simulink model "pll_type2_noise"  (Simulink 6.6)
settings: Solver=VariableStepDiscrete  StartTime=0.0  StopTime=150  RelTol=1e-3
PreLoadFcn:
  | Fs = 1000;
StopFcn:
  | figure(17)
  | hold off
  | plot(Vss_nom,'b');
  | hold on
  | plot(Vss,'r');
  | legend('Centre SS', 'Adj. SS',0);
  | 
  | doFFTplot(Fs, [Vref(round(length(Vref)*0.9):end), Vsyn(round(length(Vsyn)*0.9):end)], ['Input'; 'Synth'], 1, 18, 'hann');
  | 
  | 
  | figure(19)
  | hold off
  | plot(Vref,'b-o');
  | hold on
  | plot(Vsyn,'r-o');
  | plot(zeros(1,length(Vref)),'k--');
  | axis([0 length(Vref) -(max(abs(Vref))*1.2) (max(abs(Vref))*1.2)]);
  | legend('Input','Output',1)
libraries: xbsIndex_r4 x19, dspsrcs4 x1, simulink x1
settings Model: Creator=lcrockett  LastModifiedBy=lcrockett

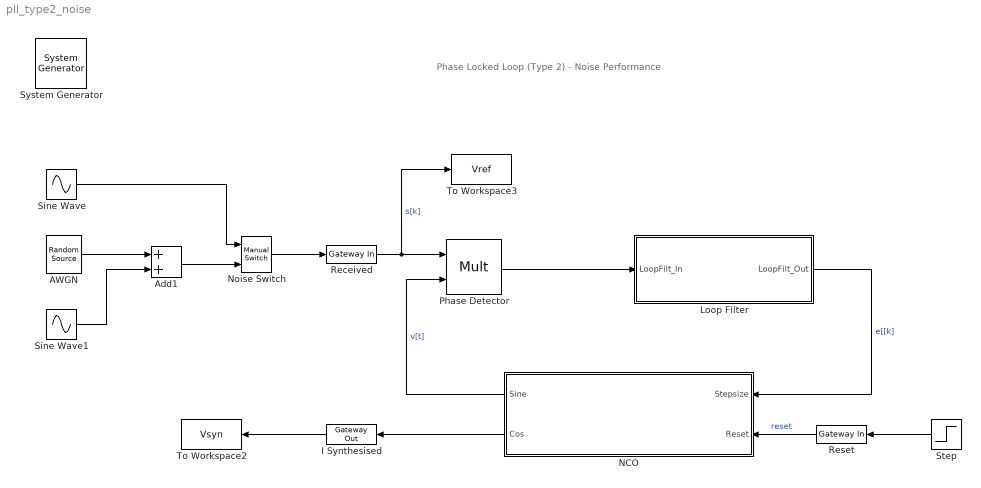
== system pll_type2_noise ==
  note: Phase Locked Loop (Type 2) - Noise Performance
  " System Generator" : xbsIndex_r4/ System Generator  Tag=genX  SystemSampleTime=-1  xilinxfamily=virtex4  part=xc4vsx35  speed=-10  package=ff668  synthesis_tool=XST  clock_wrapper=Clock Enables  directory=./netlist  testbench=off  simulink_period=1/Fs  sysclk_period=10  dcm_input_clock_period=100  incr_netlist=off  trim_vbits=Everywhere in SubSystem  dbl_ovrd=According to Block Masks  core_generation=According to Block Masks  run_coregen=off  deprecated_control=off  eval_field=0  block_type=sysgen
      settings: block_version=9.2.01
  AWGN : dspsrcs4/Random Source  SrcType=Gaussian  NormMethod=Ziggurat  CltLength=12  MinVal=0  MaxVal=1  MeanVal=0  VarVal=0.02  RepMode=Not repeatable  rawSeed=1  IsInherit=off  SampMode=Discrete  SampTime=1/Fs  SampFrame=1  DataType=Double  OutComplex=Real
  Add1 : Sum  OutScaling=2^-10
  I Synthesised : xbsIndex_r4/Gateway Out  Orientation=left  hdl_port=on  timing_constraint=None  locs_specified=off  LOCs={}  block_type=gatewayout
      settings: infoedit="Gateway out block.  Converts Xilinx fixed point inputs into ouputs of type Simulink integer, double, or fixed point.<P><P>Hardware notes:  In hardware these blocks become top level output ports or are discarded, depending on how they are configured."  block_version=9.2.01
  Loop Filter : Subsystem  mask(Loop Filter Parameters){alpha_n=2, beta_n=6, phase_det_word=32, acc_ibits=10}
      mask prompts: alpha_n "Alpha (bits to shift right by)"; beta_n "Beta (bits to shift right by)"; phase_det_word "Input wordlength"; acc_ibits "Accumulator integer bits"
      mask help:
      | The loop filter contains two paths: a proportional path and an integral path. These have coefficients Alpha and Beta, respectively.
      |
      | The wordlengths at the outputs of the shifts are extended by the degrees of the shifts. This also defines the number of fractional bits required in the accumulator of the integrator. The number of whole bits should be sufficient to prevent overflow.
      mask init:
      | alpha_shift_wl = phase_det_word + alpha_n;
      | beta_shift_wl = phase_det_word + beta_n;
  NCO : Subsystem  Orientation=left  mask(Numerically Controlled Oscillator){N=1024, LUT_w=16, F_res=0.00001, F_nom=36.7, F_s=Fs}
      mask prompts: N "Lookup Table size, N (where N = 2^n)"; LUT_w "Lookup Table output wordlength"; F_res "Desired Frequency Resolution (Hz)"; F_nom "Desired Nominal frequency (Hz)"; F_s "Sampling frequency (Hz)"
      mask help: When specifying the resolution, ensure that the required number of fractional bits are available on the input data path (which provides the step size). Otherwise, the level of frequency resolution stated on the NCO block will not be realised.
      mask init:
      | delta_mu_des = (F_res * N) / F_s;
      | fract_bits = ceil(abs((log(delta_mu_des) / log(2))));
      | whole_bits = round(log(N)/log(2));
      | mu_nom = (F_nom * N) / F_s;
      | F_res_act = F_s / ((2^fract_bits) * N);
      mask Display: fprintf(['Actual Frequency Resolution = ', num2str(F_res_act), 'Hz\n Whole Bits = ', num2str(whole_bits), '\n Fractional Bits = ', num2str(fract_bits)],'texmode','on');
  Noise Switch : simulink/Signal Routing/Manual Switch  SystemSampleTime=-1  sw=1  action=0  varsize=off
  Phase Detector : xbsIndex_r4/Mult  precision=Full  arith_type="Signed  (2's comp)"  n_bits=16  bin_pt=14  quantization=Truncate  overflow=Wrap  en=off  latency=0  dbl_ovrd=off  use_behavioral_HDL=off  use_embedded=on  opt=Speed  optimum_pipeline=off  pipeline=on  use_rpm=on  placement_style=Triangular  block_type=mult
      settings: infoedit=Hardware notes: To use the internal pipeline stage of the dedicated multiplier you must select 'Pipeline for maximum performance'.  block_version=9.2.01
  Received : xbsIndex_r4/Gateway In  arith_type="Signed  (2's comp)"  n_bits=16  bin_pt=14  quantization="Round  (unbiased: +/- Inf)"  overflow=Saturate  period=1/Fs  dbl_ovrd=off  timing_constraint=None  locs_specified=off  LOCs={}  block_type=gatewayin
      settings: infoedit="Gateway in block.  Converts inputs of type Simulink integer, double and fixed point to  Xilinx fixed point type.<P><P>Hardware notes:  In hardware these blocks become top level input ports."  block_version=9.2.01
  Reset : xbsIndex_r4/Gateway In  Orientation=left  arith_type=Boolean  n_bits=16  bin_pt=14  quantization="Round  (unbiased: +/- Inf)"  overflow=Saturate  period=1/Fs  dbl_ovrd=off  timing_constraint=None  locs_specified=off  LOCs={}  block_type=gatewayin
      settings: infoedit="Gateway in block.  Converts inputs of type Simulink integer, double and fixed point to  Xilinx fixed point type.<P><P>Hardware notes:  In hardware these blocks become top level input ports."  block_version=9.2.01
  Sine Wave : Sin  Frequency=2*pi*36  SampleTime=1/Fs
  Sine Wave1 : Sin  Amplitude=0.75  Frequency=2*pi*36  SampleTime=1/Fs
  Step : Step  Orientation=left  Time=0.1  Before=1  After=0  SampleTime=1/1000
  To Workspace2 : ToWorkspace  VariableName=Vsyn  SampleTime=-1  SaveFormat=Array
  To Workspace3 : ToWorkspace  VariableName=Vref  SampleTime=-1  SaveFormat=Array
  wires:
  NCO/1(Sine) -> Phase Detector/2  "v[t]"
  Step/1 -> Reset/1
  Reset/1 -> NCO/2(Reset)  "reset"
  Received/1 -> To Workspace3/1, Phase Detector/1  "s[k]"
  Noise Switch/1 -> Received/1
  Add1/1 -> Noise Switch/2
  Phase Detector/1 -> Loop Filter/1(LoopFilt_In)
  NCO/2(Cos) -> I Synthesised/1
  I Synthesised/1 -> To Workspace2/1
  Sine Wave/1 -> Noise Switch/1
  Loop Filter/1(LoopFilt_Out) -> NCO/1(Stepsize)  "e[[k]"
  AWGN/1 -> Add1/1
  Sine Wave1/1 -> Add1/2

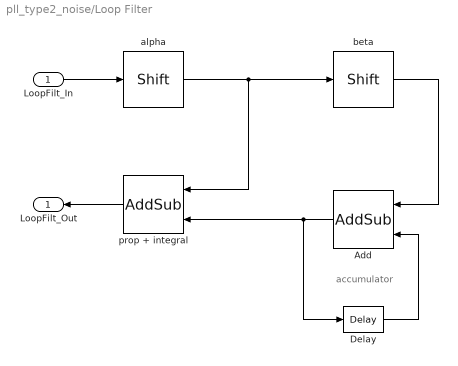
== system pll_type2_noise/Loop Filter ==
  note: accumulator
  LoopFilt_In : Inport
  Add : xbsIndex_r4/AddSub  Orientation=left  mode=Addition  use_carryin=off  use_carryout=off  en=off  latency=0  precision=User Defined  arith_type="Signed  (2's comp)"  n_bits=acc_ibits+beta_shift_wl-2  bin_pt=beta_shift_wl-2  quantization="Round  (unbiased: +/- Inf)"  overflow=Wrap  dbl_ovrd=off  use_behavioral_HDL=off  pipelined=off  use_rpm=on  block_type=addsub
      settings: block_version=9.2.01
  Delay : xbsIndex_r4/Delay  en=off  latency=1  dbl_ovrd=off  reg_retiming=off  block_type=delay
      settings: block_version=9.2.01
  alpha : xbsIndex_r4/Shift  shift_dir=Right  shift_bits=alpha_n  en=off  latency=0  precision=User Defined  arith_type="Signed  (2's comp)"  n_bits=alpha_shift_wl  bin_pt=alpha_shift_wl-2  quantization=Truncate  overflow=Wrap  dbl_ovrd=off  block_type=shift
      settings: block_version=9.2.01
  beta : xbsIndex_r4/Shift  shift_dir=Right  shift_bits=beta_n  en=off  latency=0  precision=User Defined  arith_type="Signed  (2's comp)"  n_bits=beta_shift_wl  bin_pt=beta_shift_wl-2  quantization=Truncate  overflow=Wrap  dbl_ovrd=off  block_type=shift
      settings: block_version=9.2.01
  prop + integral : xbsIndex_r4/AddSub  Orientation=left  mode=Addition  use_carryin=off  use_carryout=off  en=off  latency=0  precision=Full  arith_type="Signed  (2's comp)"  n_bits=20  bin_pt=14  quantization="Round  (unbiased: +/- Inf)"  overflow=Wrap  dbl_ovrd=off  use_behavioral_HDL=off  pipelined=off  use_rpm=on  block_type=addsub
      settings: block_version=9.2.01
  LoopFilt_Out : Outport  Orientation=left
  wires:
  Add/1 -> Delay/1, prop + integral/2
  Delay/1 -> Add/2
  LoopFilt_In/1 -> alpha/1
  prop + integral/1 -> LoopFilt_Out/1
  alpha/1 -> prop + integral/1, beta/1
  beta/1 -> Add/1

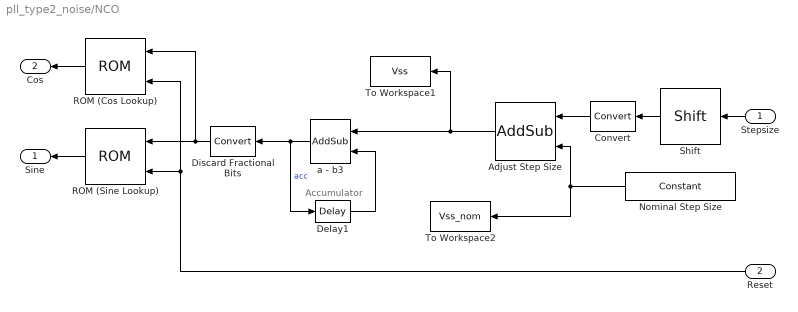
== system pll_type2_noise/NCO ==
  note: Accumulator
  Stepsize : Inport  Orientation=left
  Reset : Inport  Orientation=left  Port=2
  Adjust Step Size : xbsIndex_r4/AddSub  Orientation=left  mode=Addition  use_carryin=off  use_carryout=off  en=off  latency=0  precision=User Defined  arith_type=Unsigned  n_bits=whole_bits + fract_bits  bin_pt=fract_bits  quantization="Round  (unbiased: +/- Inf)"  overflow=Wrap  dbl_ovrd=off  use_behavioral_HDL=off  pipelined=off  use_rpm=on  block_type=addsub
      settings: block_version=9.2.01
  Convert : xbsIndex_r4/Convert  Orientation=left  arith_type="Signed  (2's comp)"  n_bits=whole_bits+fract_bits  bin_pt=fract_bits  quantization=Truncate  overflow=Wrap  latency=0  dbl_ovrd=off  pipeline=off  block_type=convert
      settings: block_version=9.2.01
  Delay1 : xbsIndex_r4/Delay  en=off  latency=1  dbl_ovrd=off  reg_retiming=off  block_type=delay
      settings: block_version=9.2.01
  Discard Fractional Bits : xbsIndex_r4/Convert  Orientation=left  arith_type=Unsigned  n_bits=whole_bits  bin_pt=0  quantization=Truncate  overflow=Wrap  latency=0  dbl_ovrd=off  pipeline=off  block_type=convert
      settings: block_version=9.2.01
  Nominal Step Size : xbsIndex_r4/Constant  Orientation=left  arith_type=Unsigned  const=mu_nom  n_bits=whole_bits + fract_bits  bin_pt=fract_bits  explicit_period=on  period=1/Fs  equ=P=C  opselect=C  inp2=PCIN>>17  opr=+  inp1=P  carry=CIN  dbl_ovrd=off  block_type=constant
      settings: block_version=9.2.01
  ROM (Cos Lookup) : xbsIndex_r4/ROM  Orientation=left  depth=N  initVector=-cos(pi*(0:(N-1))/(N/2))  distributed_mem=Block RAM  rst=on  init_reg=1  en=off  latency=1  arith_type="Signed  (2's comp)"  n_bits=LUT_w  bin_pt=LUT_w - 2  dbl_ovrd=off  optimize=Area  use_rpm=on  block_type=sprom
      settings: block_version=9.2.01
  ROM (Sine Lookup) : xbsIndex_r4/ROM  Orientation=left  depth=N  initVector=sin(pi*(0:(N-1))/(N/2))  distributed_mem=Block RAM  rst=on  init_reg=1  en=off  latency=1  arith_type="Signed  (2's comp)"  n_bits=LUT_w  bin_pt=LUT_w - 2  dbl_ovrd=off  optimize=Area  use_rpm=on  block_type=sprom
      settings: block_version=9.2.01
  Shift : xbsIndex_r4/Shift  Orientation=left  shift_dir=Left  shift_bits=4  en=off  latency=0  precision=Full  arith_type="Signed  (2's comp)"  n_bits=16  bin_pt=14  quantization=Truncate  overflow=Wrap  dbl_ovrd=off  block_type=shift
      settings: block_version=9.2.01
  To Workspace1 : ToWorkspace  VariableName=Vss  SampleTime=-1  SaveFormat=Array
  To Workspace2 : ToWorkspace  VariableName=Vss_nom  SampleTime=-1  SaveFormat=Array
  a - b3 : xbsIndex_r4/AddSub  Orientation=left  mode=Addition  use_carryin=off  use_carryout=off  en=off  latency=0  precision=User Defined  arith_type=Unsigned  n_bits=whole_bits + fract_bits  bin_pt=fract_bits  quantization=Truncate  overflow=Wrap  dbl_ovrd=off  use_behavioral_HDL=off  pipelined=off  use_rpm=on  block_type=addsub
      settings: block_version=9.2.01
  Sine : Outport  Orientation=left
  Cos : Outport  Orientation=left  Port=2
  wires:
  a - b3/1 -> Delay1/1, Discard Fractional Bits/1  "acc"
  Delay1/1 -> a - b3/2
  Discard Fractional Bits/1 -> ROM (Sine Lookup)/1, ROM (Cos Lookup)/1
  ROM (Sine Lookup)/1 -> Sine/1
  Stepsize/1 -> Shift/1
  Reset/1 -> ROM (Sine Lookup)/2, ROM (Cos Lookup)/2
  Adjust Step Size/1 -> a - b3/1, To Workspace1/1
  Nominal Step Size/1 -> Adjust Step Size/2, To Workspace2/1
  ROM (Cos Lookup)/1 -> Cos/1
  Shift/1 -> Convert/1
  Convert/1 -> Adjust Step Size/1
